simulink model "floor_versus_round"  (R2018a)
settings: Solver=FixedStepDiscrete  StartTime=0.0  StopTime=100  RelTol=1e-3
libraries: dspstat3 x6
settings Model: DataTypeOverride=Off  Creator=jonathan  LastModifiedBy=rodralez
settings DataIOCC: SaveOutput=off  SaveTime=off
settings OptimizationCC: BlockReduction=off  ConditionallyExecuteInputs=off  DefaultParameterBehavior=Inlined
settings DebuggingCC: AlgebraicLoopMsg=error  SingleTaskRateTransMsg=error  ParameterPrecisionLossMsg=none  StrictBusMsg=ErrorOnBusTreatedAsVector
settings HardwareCC: ProdBitPerPointer=32  ProdBitPerSizeT=32  ProdBitPerPtrDiffT=32  ProdLargestAtomicFloat=None  ProdIntDivRoundTo=Undefined  ProdEndianess=Unspecified  ProdWordSize=32  ProdHWDeviceType=ASIC/FPGA->ASIC/FPGA  ProdEqTarget=off
settings CodeAppCC: StateflowObjectComments=on

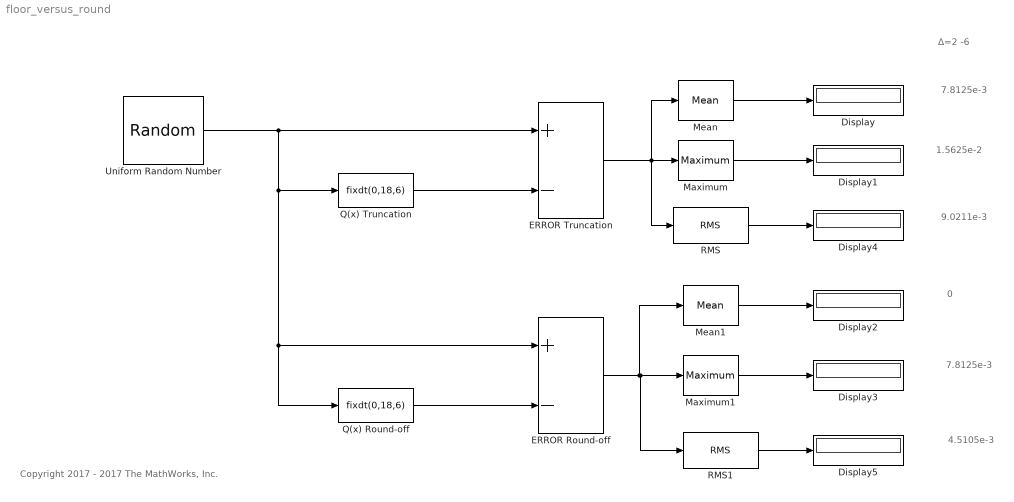
== system floor_versus_round ==
  note: Copyright 2017 - 2017 The MathWorks, Inc.
  note: 4.5105e-3
  note: 0
  note: 7.8125e-3
  note: Δ=2 -6
  note: 1.5625e-2
  note: 9.0211e-3
  note: 7.8125e-3
  Display{,1..5} (6 alike) : Display
      settings: Format=short_e
  "ERROR Round-off " : Sum  Inputs=+-
  ERROR Truncation : Sum  Inputs=+-
  Maximum : dspstat3/Maximum  operation=maximum  fcn=Running  indexBase=One  operateOver=Each column  Dimension=1  reset=None  roiEnable=off  roiType=Rectangles  roiPortion=Entire ROI  roiOutput=Individual statistics for each ROI  roiFlag=off  roundingMode=Floor  overflowMode=off  accumDataTypeStr=Inherit: Same as product output  accumLastDataTypeStr=Inherit: Same as product output
  Maximum1 : dspstat3/Maximum  operation=maximum  fcn=Running  indexBase=One  operateOver=Each column  Dimension=1  reset=None  roiEnable=off  roiType=Rectangles  roiPortion=Entire ROI  roiOutput=Individual statistics for each ROI  roiFlag=off  roundingMode=Floor  overflowMode=off  accumDataTypeStr=Inherit: Same as product output  accumLastDataTypeStr=Inherit: Same as product output
  Mean : dspstat3/Mean  run=on  reset_popup=None  directionMode=Each column  dimension=1  roiEnable=off  roiType=Rectangles  roiPortion=Entire ROI  roiOutput=Individual statistics for each ROI  roiFlag=off  roundingMode=Floor  overflowMode=off  outputDataTypeStr=Inherit: Same as accumulator  outputMin=[]  outputMax=[]  outputLastDataTypeStr=Inherit: Same as accumulator
  Mean1 : dspstat3/Mean  run=on  reset_popup=None  directionMode=Each column  dimension=1  roiEnable=off  roiType=Rectangles  roiPortion=Entire ROI  roiOutput=Individual statistics for each ROI  roiFlag=off  roundingMode=Floor  overflowMode=off  outputDataTypeStr=Inherit: Same as accumulator  outputMin=[]  outputMax=[]  outputLastDataTypeStr=Inherit: Same as accumulator
  Q(x) Round-off : DataTypeConversion  OutDataTypeStr=fixdt(0,18,6)  RndMeth=Round
  Q(x) Truncation : DataTypeConversion  OutDataTypeStr=fixdt(0,18,6)
  RMS : dspstat3/RMS  run=on  directionMode=Each column  dimension=1  reset_popup=None
  RMS1 : dspstat3/RMS  run=on  directionMode=Each column  dimension=1  reset_popup=None
  Uniform Random Number : UniformRandomNumber  Minimum=0  Maximum=100  SampleTime=0.1
  wires:
  Uniform Random Number/1 -> Q(x) Truncation/1, "ERROR Round-off "/1, Q(x) Round-off/1, ERROR Truncation/1
  Q(x) Truncation/1 -> ERROR Truncation/2
  Q(x) Round-off/1 -> "ERROR Round-off "/2
  ERROR Truncation/1 -> RMS/1, Mean/1, Maximum/1
  Mean/1 -> Display/1
  Maximum/1 -> Display1/1
  "ERROR Round-off "/1 -> Mean1/1, RMS1/1, Maximum1/1
  Mean1/1 -> Display2/1
  Maximum1/1 -> Display3/1
  RMS/1 -> Display4/1
  RMS1/1 -> Display5/1
